simulink model "pykesimulink"  (R2023b)
settings: Solver=VariableStepAuto  StartTime=0.0  StopTime=10.0  RelTol=1e-3
values from neighbouring files (symbols this model uses):
  ke0 = mean(ke)    [caracterizador.m]
  p0 = mean(p)    [caracterizador.m]
settings Model: Creator=erwinplanck  LastModifiedBy=erwinplanck

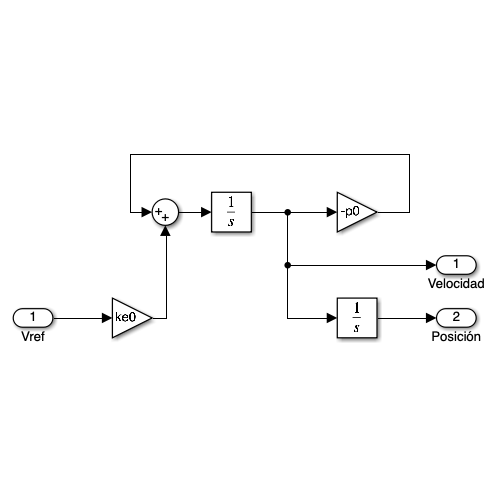
[thumbnail: Simulink's stored preview of the top-level diagram]
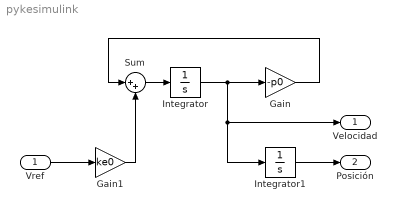
== system pykesimulink ==
  Vref : Inport
  Gain : Gain  Gain=-p0
  Gain1 : Gain  Gain=ke0
  Integrator : Integrator
  Integrator1 : Integrator
  Sum : Sum  Inputs=|++
  Velocidad : Outport
  Posición : Outport  Port=2
  wires:
  Integrator/1 -> Gain/1, Integrator1/1, Velocidad/1
  Integrator1/1 -> Posición/1
  Vref/1 -> Gain1/1
  Sum/1 -> Integrator/1
  Gain1/1 -> Sum/2
  Gain/1 -> Sum/1
